simulink library "px4_lib"  (R2025b)
settings: Solver=VariableStepAuto  StartTime=0.0  StopTime=10.0  RelTol=1e-3
undefined symbols (not defined in the file or in its folder): SampleTime
settings Model: Creator=jack  LastModifiedBy=jack
settings SFSimCC: SimCustomHeaderCode="#include \"px4_simulink_api.h\""  SimUserSources=px4_simulink_api.cpp  SimTargetLang=C++  SimDLTargetLibrary=mkl-dnn
settings RTWCC: RTWUseSimCustomCode=on  CustomHeaderCode="#include \"px4_simulink_api.h\""  CustomSource=px4_simulink_api.cpp

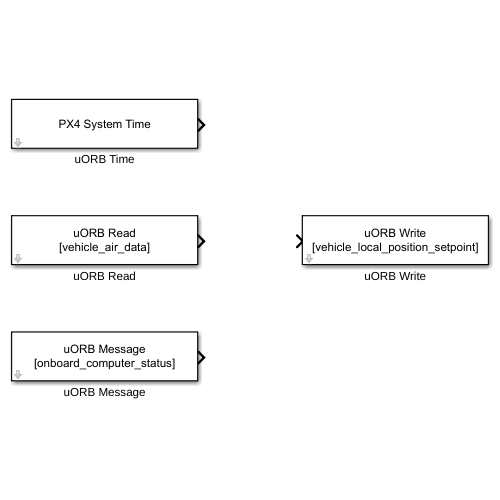
[thumbnail: Simulink's stored preview of the top-level diagram]
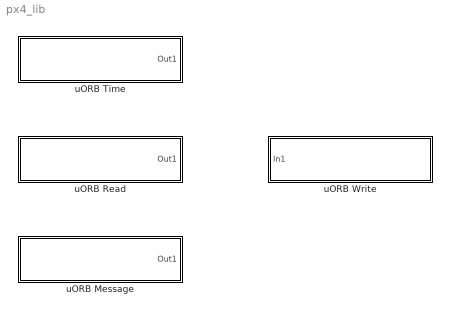
== system px4_lib ==
  uORB Message : Subsystem  mask{uorb_topic=onboard_computer_status, sample_time=-1, init_value=0}
      mask prompts: uorb_topic "uORB Topic Name"; sample_time "Sample time (-1 for inherited)"; init_value "Initialize fields to:"
      mask TypeOptions uorb_topic: action_request | actuator_armed | actuator_controls_status | actuator_outputs | actuator_servos_trim | actuator_test | adc_report | airspeed | airspeed_wind | autotune_attitude_control_status | battery_info | button_event | camera_capture | camera_status | camera_trigger | can_interface_status | cellular_status | collision_constraints | control_allocator_status | cpuload | dataman_request | dataman_response | debug_array | debug_key_value | debug_value | debug_vect | differential_pressure | distance_sensor | distance_sensor_mode_change_request | dronecan_node_status | ekf2timestamps | esc_report | esc_status | estimator_aid_source1d | estimator_aid_source2d | estimator_aid_source3d | estimator_bias | estimator_bias3d | estimator_event_flags | estimator_gps_status | estimator_innovations | estimator_selector_status | estimator_sensor_bias | estimator_states | estimator_status | estimator_status_flags | failsafe_flags | failure_detector_status | figure_eight_status | fixed_wing_lateral_guidance_status | fixed_wing_lateral_status | fixed_wing_runway_control | flight_phase_estimation | follow_target | follow_target_estimator | follow_target_status | fuel_tank_status | generator_status | geofence_result | geofence_status | gimbal_controls | gimbal_device_attitude_status | gimbal_device_information | gimbal_device_set_attitude | gimbal_manager_information | gimbal_manager_set_attitude | gimbal_manager_set_manual_control | gimbal_manager_status | gpio_config | gpio_in | gpio_out | gpio_request | gps_dump | gps_inject_data | gripper | health_report | heater_status | hover_thrust_estimate | input_rc | internal_combustion_engine_control | internal_combustion_engine_status | iridiumsbd_status | irlock_report | landing_gear | landing_gear_wheel | landing_target_innovations | landing_target_pose | launch_detection_status | led_control | log_message | logger_status | mag_worker_data | magnetometer_bias_estimate | manual_control_switches | mavlink_log | mavlink_tunnel | message_format_request | message_format_response | mission | mission_result | mount_orientation | navigator_mission_item | navigator_status | neural_control | normalized_unsigned_setpoint | obstacle_distance | offboard_control_mode | onboard_computer_status | open_drone_id_arm_status | open_drone_id_operator_id | open_drone_id_self_id | open_drone_id_system | orb_test | orb_test_large | orb_test_medium | orbit_status | parameter_reset_request | parameter_set_used_request | parameter_set_value_request | parameter_set_value_response | parameter_update | ping | position_controller_landing_status | position_controller_status | position_setpoint | position_setpoint_triplet | power_button_state | power_monitor | pps_capture | pure_pursuit_status | pwm_input | px4io_status | qshell_req | qshell_retval | radio_status | rate_ctrl_status | rc_channels | rc_parameter_map | rover_attitude_setpoint | rover_attitude_status | rover_position_setpoint | rover_rate_setpoint | rover_rate_status | rover_speed_setpoint | rover_speed_status | rover_steering_setpoint | rover_throttle_setpoint | rpm | rtl_status | rtl_time_estimate | satellite_info | sensor_accel | sensor_accel_fifo | sensor_airflow | sensor_baro | sensor_combined | sensor_correction | sensor_gnss_relative | sensor_gnss_status | sensor_gps | sensor_gyro | sensor_gyro_fft | sensor_gyro_fifo | sensor_hygrometer | sensor_mag | sensor_optical_flow | sensor_preflight_mag | sensor_selection | sensor_uwb | sensors_status | sensors_status_imu | system_power | takeoff_status | task_stack_info | tecs_status | telemetry_status | tiltrotor_extra_controls | timesync_status | trajectory_setpoint6dof | transponder_report | tune_control | uavcan_parameter_request | uavcan_parameter_value | ulog_stream | ulog_stream_ack | vehicle_acceleration | vehicle_air_data | vehicle_angular_acceleration_setpoint | vehicle_constraints | vehicle_imu | vehicle_imu_status | vehicle_local_position_setpoint | vehicle_magnetometer | vehicle_optical_flow | vehicle_optical_flow_vel | vehicle_roi | vehicle_thrust_setpoint | vehicle_torque_setpoint | velocity_limits | wheel_encoders | yaw_estimator_status
      mask TypeOptions init_value: NaN | 0
      mask Display: fprintf('uORB Message\n[%s]',get_param(gcb, 'uorb_topic'));
  uORB Read : Subsystem  mask{uorb_topic=vehicle_air_data, sample_time=-1}
      mask prompts: uorb_topic "uORB Topic Name"; sample_time "Sample time (-1 for inherited)"
      mask TypeOptions uorb_topic: action_request | actuator_armed | actuator_controls_status | actuator_outputs | actuator_servos_trim | actuator_test | adc_report | airspeed | airspeed_wind | autotune_attitude_control_status | battery_info | button_event | camera_capture | camera_status | camera_trigger | can_interface_status | cellular_status | collision_constraints | control_allocator_status | cpuload | dataman_request | dataman_response | debug_array | debug_key_value | debug_value | debug_vect | differential_pressure | distance_sensor | distance_sensor_mode_change_request | dronecan_node_status | ekf2timestamps | esc_report | esc_status | estimator_aid_source1d | estimator_aid_source2d | estimator_aid_source3d | estimator_bias | estimator_bias3d | estimator_event_flags | estimator_gps_status | estimator_innovations | estimator_selector_status | estimator_sensor_bias | estimator_states | estimator_status | estimator_status_flags | failsafe_flags | failure_detector_status | figure_eight_status | fixed_wing_lateral_guidance_status | fixed_wing_lateral_status | fixed_wing_runway_control | flight_phase_estimation | follow_target | follow_target_estimator | follow_target_status | fuel_tank_status | generator_status | geofence_result | geofence_status | gimbal_controls | gimbal_device_attitude_status | gimbal_device_information | gimbal_device_set_attitude | gimbal_manager_information | gimbal_manager_set_attitude | gimbal_manager_set_manual_control | gimbal_manager_status | gpio_config | gpio_in | gpio_out | gpio_request | gps_dump | gps_inject_data | gripper | health_report | heater_status | hover_thrust_estimate | input_rc | internal_combustion_engine_control | internal_combustion_engine_status | iridiumsbd_status | irlock_report | landing_gear | landing_gear_wheel | landing_target_innovations | landing_target_pose | launch_detection_status | led_control | log_message | logger_status | mag_worker_data | magnetometer_bias_estimate | manual_control_switches | mavlink_log | mavlink_tunnel | message_format_request | message_format_response | mission | mission_result | mount_orientation | navigator_mission_item | navigator_status | neural_control | normalized_unsigned_setpoint | obstacle_distance | offboard_control_mode | onboard_computer_status | open_drone_id_arm_status | open_drone_id_operator_id | open_drone_id_self_id | open_drone_id_system | orb_test | orb_test_large | orb_test_medium | orbit_status | parameter_reset_request | parameter_set_used_request | parameter_set_value_request | parameter_set_value_response | parameter_update | ping | position_controller_landing_status | position_controller_status | position_setpoint | position_setpoint_triplet | power_button_state | power_monitor | pps_capture | pure_pursuit_status | pwm_input | px4io_status | qshell_req | qshell_retval | radio_status | rate_ctrl_status | rc_channels | rc_parameter_map | rover_attitude_setpoint | rover_attitude_status | rover_position_setpoint | rover_rate_setpoint | rover_rate_status | rover_speed_setpoint | rover_speed_status | rover_steering_setpoint | rover_throttle_setpoint | rpm | rtl_status | rtl_time_estimate | satellite_info | sensor_accel | sensor_accel_fifo | sensor_airflow | sensor_baro | sensor_combined | sensor_correction | sensor_gnss_relative | sensor_gnss_status | sensor_gps | sensor_gyro | sensor_gyro_fft | sensor_gyro_fifo | sensor_hygrometer | sensor_mag | sensor_optical_flow | sensor_preflight_mag | sensor_selection | sensor_uwb | sensors_status | sensors_status_imu | system_power | takeoff_status | task_stack_info | tecs_status | telemetry_status | tiltrotor_extra_controls | timesync_status | trajectory_setpoint6dof | transponder_report | tune_control | uavcan_parameter_request | uavcan_parameter_value | ulog_stream | ulog_stream_ack | vehicle_acceleration | vehicle_air_data | vehicle_angular_acceleration_setpoint | vehicle_constraints | vehicle_imu | vehicle_imu_status | vehicle_local_position_setpoint | vehicle_magnetometer | vehicle_optical_flow | vehicle_optical_flow_vel | vehicle_roi | vehicle_thrust_setpoint | vehicle_torque_setpoint | velocity_limits | wheel_encoders | yaw_estimator_status
      mask Display: fprintf('uORB Read\n[%s]',get_param(gcb, 'uorb_topic'));
  uORB Time : Subsystem  mask{sample_time=-1}
      mask prompts: sample_time "Sample time (-1 for inherited)"
      mask Display: disp('PX4 System Time');
  uORB Write : Subsystem  mask{uorb_topic=vehicle_local_position_setpoint, sample_time=-1}
      mask prompts: uorb_topic "uORB Topic Name"; sample_time "Sample time (-1 for inherited)"
      mask TypeOptions uorb_topic: action_request | actuator_armed | actuator_controls_status | actuator_outputs | actuator_servos_trim | actuator_test | adc_report | airspeed | airspeed_wind | autotune_attitude_control_status | battery_info | button_event | camera_capture | camera_status | camera_trigger | can_interface_status | cellular_status | collision_constraints | control_allocator_status | cpuload | dataman_request | dataman_response | debug_array | debug_key_value | debug_value | debug_vect | differential_pressure | distance_sensor | distance_sensor_mode_change_request | dronecan_node_status | ekf2timestamps | esc_report | esc_status | estimator_aid_source1d | estimator_aid_source2d | estimator_aid_source3d | estimator_bias | estimator_bias3d | estimator_event_flags | estimator_gps_status | estimator_innovations | estimator_selector_status | estimator_sensor_bias | estimator_states | estimator_status | estimator_status_flags | failsafe_flags | failure_detector_status | figure_eight_status | fixed_wing_lateral_guidance_status | fixed_wing_lateral_status | fixed_wing_runway_control | flight_phase_estimation | follow_target | follow_target_estimator | follow_target_status | fuel_tank_status | generator_status | geofence_result | geofence_status | gimbal_controls | gimbal_device_attitude_status | gimbal_device_information | gimbal_device_set_attitude | gimbal_manager_information | gimbal_manager_set_attitude | gimbal_manager_set_manual_control | gimbal_manager_status | gpio_config | gpio_in | gpio_out | gpio_request | gps_dump | gps_inject_data | gripper | health_report | heater_status | hover_thrust_estimate | input_rc | internal_combustion_engine_control | internal_combustion_engine_status | iridiumsbd_status | irlock_report | landing_gear | landing_gear_wheel | landing_target_innovations | landing_target_pose | launch_detection_status | led_control | log_message | logger_status | mag_worker_data | magnetometer_bias_estimate | manual_control_switches | mavlink_log | mavlink_tunnel | message_format_request | message_format_response | mission | mission_result | mount_orientation | navigator_mission_item | navigator_status | neural_control | normalized_unsigned_setpoint | obstacle_distance | offboard_control_mode | onboard_computer_status | open_drone_id_arm_status | open_drone_id_operator_id | open_drone_id_self_id | open_drone_id_system | orb_test | orb_test_large | orb_test_medium | orbit_status | parameter_reset_request | parameter_set_used_request | parameter_set_value_request | parameter_set_value_response | parameter_update | ping | position_controller_landing_status | position_controller_status | position_setpoint | position_setpoint_triplet | power_button_state | power_monitor | pps_capture | pure_pursuit_status | pwm_input | px4io_status | qshell_req | qshell_retval | radio_status | rate_ctrl_status | rc_channels | rc_parameter_map | rover_attitude_setpoint | rover_attitude_status | rover_position_setpoint | rover_rate_setpoint | rover_rate_status | rover_speed_setpoint | rover_speed_status | rover_steering_setpoint | rover_throttle_setpoint | rpm | rtl_status | rtl_time_estimate | satellite_info | sensor_accel | sensor_accel_fifo | sensor_airflow | sensor_baro | sensor_combined | sensor_correction | sensor_gnss_relative | sensor_gnss_status | sensor_gps | sensor_gyro | sensor_gyro_fft | sensor_gyro_fifo | sensor_hygrometer | sensor_mag | sensor_optical_flow | sensor_preflight_mag | sensor_selection | sensor_uwb | sensors_status | sensors_status_imu | system_power | takeoff_status | task_stack_info | tecs_status | telemetry_status | tiltrotor_extra_controls | timesync_status | trajectory_setpoint6dof | transponder_report | tune_control | uavcan_parameter_request | uavcan_parameter_value | ulog_stream | ulog_stream_ack | vehicle_acceleration | vehicle_air_data | vehicle_angular_acceleration_setpoint | vehicle_constraints | vehicle_imu | vehicle_imu_status | vehicle_local_position_setpoint | vehicle_magnetometer | vehicle_optical_flow | vehicle_optical_flow_vel | vehicle_roi | vehicle_thrust_setpoint | vehicle_torque_setpoint | velocity_limits | wheel_encoders | yaw_estimator_status
      mask Display: fprintf('uORB Write\n[%s]',get_param(gcb, 'uorb_topic'));

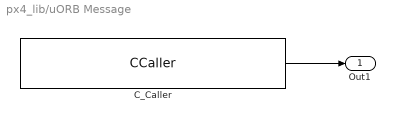
== system px4_lib/uORB Message ==
  C_Caller : CCaller  FunctionName=init_onboard_computer_status  PortSpecificationStruct="%)30     .    \" 0   8    (     @         %    \"     (    !     0         %  0 \"0    $    _    07)G3F%M90  4&]R=$YA;64 4V-O<&4     26YD97@     5'EP90      4VEZ90      27-';&]B86P   X    P    !@    @    $          4    (     0    ,    !         !   P!O=70 #@   #     &    \"     0         !0    @    !     P    $         $  # &]U=  .    .     8    (    !          %    \"     $    &     0         0    !@   $]U='!U=   #@   #@    &    \"     8         !0    @    !     0    $         \"0    @               X   !0    !@    @    $          4    (     0   !X    !         !     >    0G5S.B!O;F)O87)D7V-O;7!U=&5R7W-T871U<U]S   .    ,     8    (    !          %    \"     $    !     0         0  $ ,0    X    P    !@    @    ) @        4    (     0    $    !          (  0      #@   $@    &    \"     0         !0    @    !    $0    $         $    !$   !I;FET:6%L:7IE7W1O7VYA;@         .    2     8    (    !          %    \"     $    1     0         0    $0   &EN:71I86QI>F5?=&]?;F%N          X   !     !@    @    $          4    (     0    D    !         !     )    4&%R86UE=&5R          X    X    !@    @    &          4    (     0    $    !          D    (               .    .     8    (    !          %    \"     $    '     0         0    !P   &)O;VQE86X #@   #     &    \"     0         !0    @    !     0    $         $  ! #$    .    ,     8    (    \"0(        %    \"     $    !     0         \"  $"  SampleTime=SampleTime  initialize_to_nan=false  SampleTime=-1
  Out1 : Outport  OutDataTypeStr=Bus: onboard_computer_status_s
  wires:
  C_Caller/1 -> Out1/1

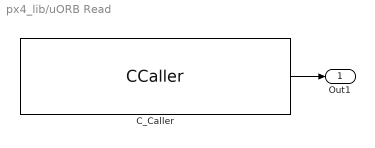
== system px4_lib/uORB Read ==
  C_Caller : CCaller  FunctionName=read_vehicle_air_data  PortSpecificationStruct="%)30     .    * (   8    (     @         %    \"     $    !     0         %  0 \"0    $    _    07)G3F%M90  4&]R=$YA;64 4V-O<&4     26YD97@     5'EP90      4VEZ90      27-';&]B86P   X    P    !@    @    $          4    (     0    ,    !         !   P!O=70 #@   #     &    \"     0         !0    @    !     P    $         $  # &]U=  .    .     8    (    !          %    \"     $    &     0         0    !@   $]U='!U=   #@   #@    &    \"     8         !0    @    !     0    $         \"0    @               X   !(    !@    @    $          4    (     0   !<    !         !     7    0G5S.B!V96AI8VQE7V%I<E]D871A7W, #@   #     &    \"     0         !0    @    !     0    $         $  ! #$    .    ,     8    (    \"0(        %    \"     $    !     0         \"  $"
  Out1 : Outport  OutDataTypeStr=Bus: vehicle_air_data_s
  wires:
  C_Caller/1 -> Out1/1

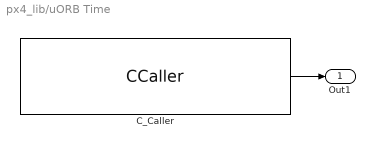
== system px4_lib/uORB Time ==
  C_Caller : CCaller  FunctionName=read_px4_system_time  PortSpecificationStruct="%)30     .    & (   8    (     @         %    \"     $    !     0         %  0 \"0    $    _    07)G3F%M90  4&]R=$YA;64 4V-O<&4     26YD97@     5'EP90      4VEZ90      27-';&]B86P   X    P    !@    @    $          4    (     0    ,    !         !   P!O=70 #@   #     &    \"     0         !0    @    !     P    $         $  # &]U=  .    .     8    (    !          %    \"     $    &     0         0    !@   $]U='!U=   #@   #@    &    \"     8         !0    @    !     0    $         \"0    @               X    X    !@    @    $          4    (     0    8    !         !     &    =6EN=#8T   .    ,     8    (    !          %    \"     $    !     0         0  $ ,0    X    P    !@    @    ) @        4    (     0    $    !          (  0"
  Out1 : Outport  OutDataTypeStr=uint64
  wires:
  C_Caller/1 -> Out1/1

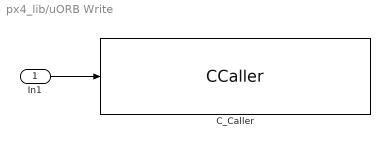
== system px4_lib/uORB Write ==
  In1 : Inport  OutDataTypeStr=Bus: vehicle_local_position_setpoint_s
  C_Caller : CCaller  FunctionName=write_vehicle_local_position_setpoint  PortSpecificationStruct="%)30     .    . (   8    (     @         %    \"     $    !     0         %  0 \"0    $    _    07)G3F%M90  4&]R=$YA;64 4V-O<&4     26YD97@     5'EP90      4VEZ90      27-';&]B86P   X    P    !@    @    $          4    (     0    (    !         !   @!I;@  #@   #     &    \"     0         !0    @    !     @    $         $  \" &EN   .    .     8    (    !          %    \"     $    %     0         0    !0   $EN<'5T    #@   #@    &    \"     8         !0    @    !     0    $         \"0    @               X   !8    !@    @    $          4    (     0   \"8    !         !     F    0G5S.B!V96AI8VQE7VQO8V%L7W!O<VET:6]N7W-E='!O:6YT7W,   X    P    !@    @    $          4    (     0    $    !         !   0 Q    #@   #     &    \"     D\"        !0    @    !     0    $          @ !"
  wires:
  In1/1 -> C_Caller/1
